simulink model "MBD_SpeedControl"  (R2024a)
settings: Solver=FixedStepDiscrete  StartTime=0.0  StopTime=20.0  RelTol=1e-3
libraries: SignalEditorBlockLib x1
settings Model: Creator=Hakima Ayed  LastModifiedBy=Hakima Ayed
settings OptimizationCC: DefaultParameterBehavior=Inlined  EnhancedBackFolding=on  PassReuseOutputArgsAs=Individual arguments  ZeroExternalMemoryAtStartup=off  ZeroInternalMemoryAtStartup=off  OptimizeBlockOrder=speed  DifferentSizesBufferReuse=on  OptimizationCustomize=off  EfficientTunableParamExpr=on
settings DebuggingCC: ParameterTunabilityLossMsg=error
settings SFSimCC: MATLABDynamicMemAlloc=off
settings RTWCC: Description=Embedded Coder  SystemTargetFile=ert.tlc  TemplateMakefile=ert_default_tmf
settings CodeAppCC: ForceParamTrailComments=on  IgnoreCustomStorageClasses=off  OperatorAnnotations=on  SimulinkDataObjDesc=on  SFDataObjDesc=on  InsertBlockDesc=on
settings ERTTargetCC: TargetLangStandard=C99 (ISO)  GenerateSampleERTMain=on  SupportContinuousTime=on  InlinedParameterPlacement=NonHierarchical  ERTCustomFileTemplate=example_file_process.tlc

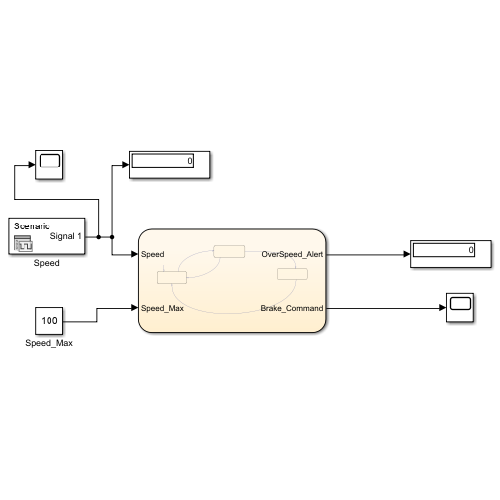
[thumbnail: Simulink's stored preview of the top-level diagram]
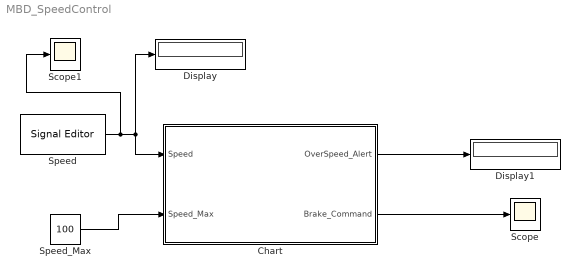
== system MBD_SpeedControl ==
  Chart : Stateflow chart  TreatAsAtomicUnit=on
  Display : Display
  Display1 : Display
  Scope : Scope
  Scope1 : Scope
  Speed : SignalEditorBlockLib/Signal Editor  FileName=C:\Users\Hakima Ayed\Desktop\Vitesse\vitesse simulé d'une voiture.mat  ActiveScenario=Scenario  ActiveSignal=Signal 1  IsBus=off  OutputBusObjectStr=Bus: BusObject  SampleTime=0  Interpolate=off  ZeroCross=off  OutputAfterFinalValue=Setting to zero  Unit=inherit  PreserveSignalName=on  ApplySigPropsToAllScenarios=on  ApplySigPropsToAllSignals=off
  Speed_Max : Constant  Value=100
  wires:
  Speed_Max/1 -> Chart/2(Speed_Max)
  Chart/1(OverSpeed_Alert) -> Display1/1
  Chart/2(Brake_Command) -> Scope/1
  Speed/1 -> Scope1/1, Display/1, Chart/1(Speed)

== stateflow chart MBD_SpeedControl/Chart ==
  state Alerte
    OverSpeed_Alert = true;
    Brake_Command = false;
  state Freinage
    OverSpeed_Alert = true;
    Brake_Command = true;
  state Normal
    OverSpeed_Alert = false;
    Brake_Command=false;
  Normal -> Alerte : [Speed > Speed_Max
      | ]
  Alerte -> Freinage [order 1] : [Speed > Speed_Max + 20
      | ]
  Alerte -> Normal [order 2] : [Speed <= Speed_Max
      | ]
  (default) -> Normal
  Freinage -> Normal : [Speed <= Speed_Max
      | ]
  data: Speed input size=1; Speed_Max input size=1; OverSpeed_Alert output boolean size=1; Brake_Command output boolean size=1
